simulink model "thermo_state_machine"  (R2024b)
settings: Solver=VariableStepAuto  StartTime=0.0  StopTime=10.0  RelTol=1e-3

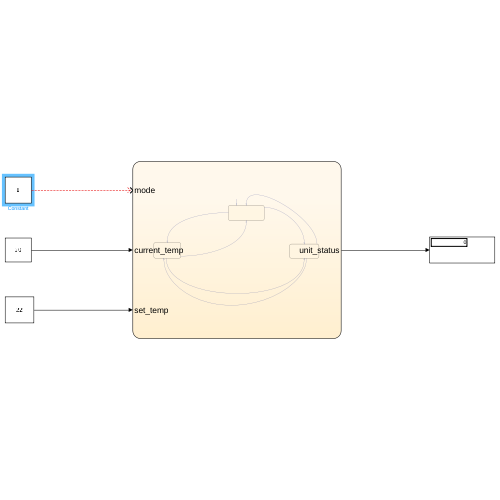
[thumbnail: Simulink's stored preview of the top-level diagram]
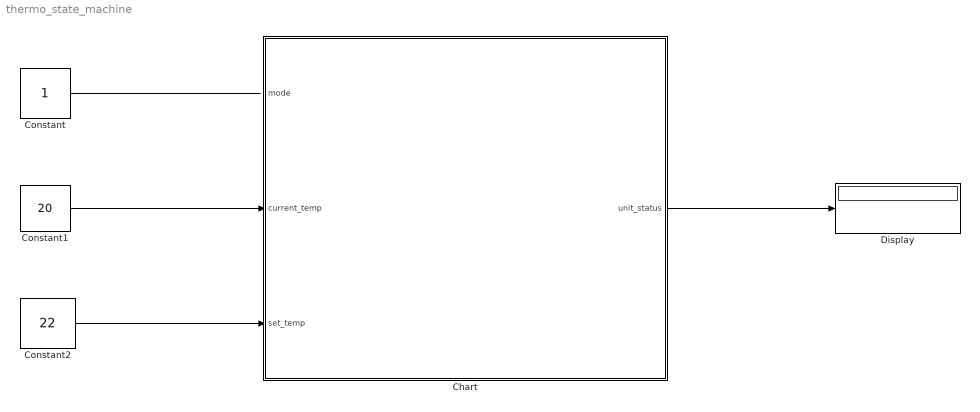
== system thermo_state_machine ==
  Chart : Stateflow chart  TreatAsAtomicUnit=on
  Constant : Constant
  Constant1 : Constant  Value=20
  Constant2 : Constant  Value=22
  Display : Display
  wires:
  Constant1/1 -> Chart/2(current_temp)
  Constant2/1 -> Chart/3(set_temp)
  Chart/1(unit_status) -> Display/1
  Constant/1 -> ?

== stateflow chart thermo_state_machine/Chart ==
  state off
    unit_status=0
  state Heating
    unit_status=1
  state Cooling
    unit_status=1
  Cooling -> off [order 1] : [mode==0]{current_temp<=set_temp}
  (default) -> off
  off -> Cooling [order 2] : [mode==2]
  off -> Heating [order 1] : [mode==1]
  Heating -> off [order 1] : [mode==0]{current_temp>=set_temp}
  Cooling -> Heating [order 2] : [mode==1]
  Heating -> Cooling [order 2] : [mode==2]
  data: mode input uint8; current_temp input double; set_temp input double; unit_status output uint8 size=1
